simulink model "AI_shema"  (Simulink 8.5)
settings: Solver=ode15s  StartTime=0.0  StopTime=1  RelTol=1e-6  AbsTol=1e-5
values from neighbouring files (symbols this model uses):
  distanca = nova_udaljenost(i)    [AI.m]
  R = novi_otpor_JKS(i)    [AI.m]
libraries: powerlib x11, powerlib_meascontrol x1
settings Model: Creator=User  LastModifiedBy=User
settings SolverCC: InitialStep=1e-6
settings DataIOCC: SignalLoggingSaveFormat=Dataset
settings OptimizationCC: ExpressionDepthLimit=128
settings DebuggingCC: UnderspecifiedInitializationDetection=Simplified  MergeDetectMultiDrivingBlocksExec=error  FcnCallInpInsideContextMsg=EnableAllAsError  StateNameClashWarn=none
settings GRTTargetCC: CombineOutputUpdateFcns=on  GRTInterface=off

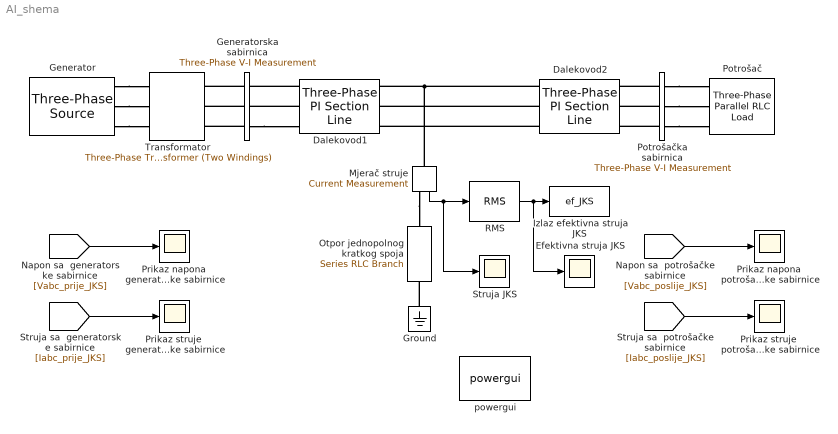
== system AI_shema ==
  Dalekovod1 : powerlib/Elements/Three-Phase PI Section Line  LConnTagsString=a|b|c  RConnTagsString=A|B|C  Frequency=50  Resistances=[ 0.01273 0.03819]  Inductances="[ 0.9337e-3  2.8011e-3]"  Capacitances=[12.74e-9 4.247e-9]  Length=distanca
  Dalekovod2 : powerlib/Elements/Three-Phase PI Section Line  LConnTagsString=a|b|c  RConnTagsString=A|B|C  Frequency=50  Resistances=[ 0.01273 0.03819]  Inductances="[ 0.9337e-3  2.8011e-3]"  Capacitances=[12.74e-9 4.247e-9]  Length=80-distanca
  Efektivna struja JKS : Scope
      settings: SaveName=ScopeData5
  "Generator " : powerlib/Electrical Sources/Three-Phase Source  Voltage=15.4e3  PhaseAngle=0  Frequency=50  InternalConnection=Yg  SpecifyImpedance=on  Resistance=0.8929  Inductance=16.58e-3  ShortCircuitLevel=250e6  BaseVoltage=15.4e3  XRratio=7  BusType=swing  Pref=0  Qref=0  Qmin=-inf  Qmax=inf
  Generatorska sabirnica : powerlib/Measurements/Three-Phase V-I Measurement  VoltageMeasurement=phase-to-ground  SetLabelV=on  LabelV=Vabc_prije_JKS  Vpu=off  VpuLL=off  CurrentMeasurement=yes  SetLabelI=on  LabelI=Iabc_prije_JKS  Ipu=off  Pbase=100e6  Vbase=500e3  OutputType=Complex  PhasorSimulation=off  PSBequivalent=0
  Ground : powerlib/Elements/Ground  LConnTagsString=a
  Izlaz efektivna struja JKS : ToWorkspace  VariableName=ef_JKS  SampleTime=-1
  Mjerač struje : powerlib/Measurements/Current Measurement  PhasorSimulation=off  OutputType=Complex  PSBequivalent=0
  Otpor jednopolnog kratkog spoja : powerlib/Elements/Series RLC Branch  LConnTagsString=__new0  RConnTagsString=__new0  BranchType=R  Resistance=R  Inductance=1e-3  SetiL0=off  InitialCurrent=0  Capacitance=1e-6  Setx0=off  InitialVoltage=0  Measurements=None
  Potrošač : powerlib/Elements/Three-Phase Parallel RLC Load  LConnTagsString=A|B|C  Configuration=Y (grounded)  NominalVoltage=110e3  NominalFrequency=50  ActivePower=2e6  InductivePower=0.2e6  CapacitivePower=0  Measurements=None  LoadType=constant Z
  Potrošačka sabirnica : powerlib/Measurements/Three-Phase V-I Measurement  VoltageMeasurement=phase-to-ground  SetLabelV=on  LabelV=Vabc_poslije_JKS  Vpu=off  VpuLL=off  CurrentMeasurement=yes  SetLabelI=on  LabelI=Iabc_poslije_JKS  Ipu=off  Pbase=100e6  Vbase=500e3  OutputType=Complex  PhasorSimulation=off  PSBequivalent=0
  Prikaz napona  generatorske sabirnice : Scope
  Prikaz napona  potrošačke sabirnice : Scope
      settings: SaveName=ScopeData2
  Prikaz struje  generatorske sabirnice : Scope
  Prikaz struje  potrošačke sabirnice : Scope
      settings: SaveName=ScopeData3
  RMS : powerlib_meascontrol/Measurements/RMS  TrueRMS=on  Freq=50  RMSInit=568  Ts=1
  Struja JKS : Scope
      settings: SaveName=ScopeData4
  Transformator : powerlib/Elements/Three-Phase Transformer (Two Windings)  Winding1Connection=Yg  Winding2Connection=Yg  CoreType=Three single-phase transformers  SetSaturation=off  Hysteresis=off  DataFile='hysteresis'  SetInitialFlux=off  Measurements=None  UNITS=pu  NominalPower=[ 25e6 , 50 ]  Winding1=[ 15.4e3 , 0.002 , 0.08 ]  Winding2=[ 110e3 , 0.002 , 0.08 ]  Rm=500  Lm=500  L0=0.5  Saturation=[ 0,0 ; 0.0024,1.2 ; 1.0,1.52 ]  InitialFluxes=[ 0.8 , -0.8 , 0.7 ]  MoreParameters=off  BreakLoop=off  DataType=off  TransfoNumber=1
  powergui : powerlib/powergui  Priority=1  SimulationMode=Continuous  SolverType=Tustin/Backward Euler (TBE)  SampleTime=50e-6  frequency=60  SPID=off  DisableSnubberDevices=off  DisableRonSwitches=off  DisableVfSwitches=off  SwTol=0  DisplayEquations=off  Interpol=off  methode=off  Ts=100  FunctionMessages=off  echomessages=off  HookPort=off  EnableUseOfTLC=off  x0status=blocks  frequencyindice=50  Pbase=100e6  ErrMax=1e-4  Iterations=50  UnitsV=kV  UnitsW=MW  buscounter=0  RestoreLinks=warning  ResistiveCurrentMeasurement=off  Frange=[0:2:500]  Ylog=off  Xlog=on  ShowGrid=off  save=off  variable=ZData  structure=0  ZoomFFT=off  StartTime=0.0  cycles=1  DisplayStyle=1  fundamental=60  FreqAxis=off  MaxFrequency=1000  frequencyindicesteady=1  RmsSteady=1  display=off
  wires:
  [Vabc_prije_JKS] -> Prikaz napona  generatorske sabirnice/1
  [Iabc_prije_JKS] -> Prikaz struje  generatorske sabirnice/1
  [Vabc_poslije_JKS] -> Prikaz napona  potrošačke sabirnice/1
  [Iabc_poslije_JKS] -> Prikaz struje  potrošačke sabirnice/1
  Mjerač struje/1 -> Struja JKS/1, RMS/1
  RMS/1 -> Efektivna struja JKS/1, Izlaz efektivna struja JKS/1
  connections:
  Dalekovod2/LConn1 -- Mjerač struje/LConn1 -- Dalekovod1/RConn1
  Dalekovod2/LConn2 -- Dalekovod1/RConn2
  Dalekovod2/LConn3 -- Dalekovod1/RConn3
  Potrošačka sabirnica/RConn1 -- Potrošač/LConn1
  Potrošačka sabirnica/RConn2 -- Potrošač/LConn2
  Potrošačka sabirnica/RConn3 -- Potrošač/LConn3
  Potrošačka sabirnica/LConn1 -- Dalekovod2/RConn1
  Potrošačka sabirnica/LConn2 -- Dalekovod2/RConn2
  Potrošačka sabirnica/LConn3 -- Dalekovod2/RConn3
  Dalekovod1/LConn1 -- Generatorska sabirnica/RConn1
  Dalekovod1/LConn2 -- Generatorska sabirnica/RConn2
  Generatorska sabirnica/RConn3 -- Dalekovod1/LConn3
  Generatorska sabirnica/LConn3 -- Transformator/RConn3
  Generatorska sabirnica/LConn2 -- Transformator/RConn2
  Generatorska sabirnica/LConn1 -- Transformator/RConn1
  "Generator "/RConn1 -- Transformator/LConn1
  "Generator "/RConn2 -- Transformator/LConn2
  "Generator "/RConn3 -- Transformator/LConn3
  Ground/LConn1 -- Otpor jednopolnog kratkog spoja/RConn1
  Mjerač struje/RConn1 -- Otpor jednopolnog kratkog spoja/LConn1
